simulink model "T2_simulation_2020a"  (R2022a)
settings: Solver=VariableStepAuto  StartTime=0.0  StopTime=simTime  RelTol=1e-3
values from neighbouring files (symbols this model uses):
  C11 = -0.1    [T2_PreLoadFcn.m]
  C21 = -0.1    [T2_PreLoadFcn.m]
undefined symbols (not defined in the file or in its folder): sysID_DAQ
libraries: cstblocks x1
settings Model: Creator=user
settings SolverCC: AlgebraicLoopSolver=TrustRegion
settings DataIOCC: ReturnWorkspaceOutputs=off
settings DebuggingCC: UnconnectedInputMsg=warning  UnconnectedOutputMsg=warning  UnconnectedLineMsg=warning  SFMachineParentedDataDiag=warning

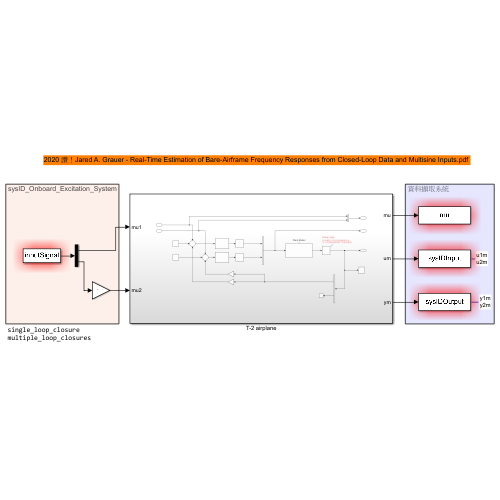
[thumbnail: Simulink's stored preview of the top-level diagram]
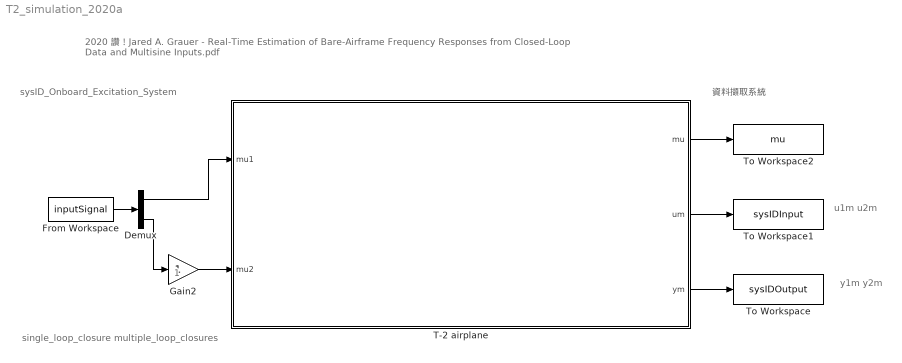
== system T2_simulation_2020a ==
  note: 1
  note: single_loop_closure
      | multiple_loop_closures
  note: sysID_Onboard_Excitation_System
  note: 資料擷取系統
  note: 2020 讚！Jared A. Grauer - Real-Time Estimation of Bare-Airframe Frequency Responses from Closed-Loop Data and Multisine Inputs.pdf
  note: u1m
      | u2m
  note: y1m
      | y2m
  Demux : Demux  Outputs=2
  From Workspace : FromWorkspace  VariableName=inputSignal  OutputAfterFinalValue=Holding final value
  Gain2 : Gain
  T-2 airplane : Subsystem
  To Workspace : ToWorkspace  VariableName=sysIDOutput  SaveFormat=Timeseries  SampleTime=sysID_DAQ.sampleTime
  To Workspace1 : ToWorkspace  VariableName=sysIDInput  SaveFormat=Timeseries  SampleTime=sysID_DAQ.sampleTime
  To Workspace2 : ToWorkspace  VariableName=mu  SaveFormat=Timeseries  SampleTime=sysID_DAQ.sampleTime
  wires:
  T-2 airplane/2(um) -> To Workspace1/1
  T-2 airplane/3(ym) -> To Workspace/1
  Gain2/1 -> T-2 airplane/2(mu2)
  Demux/2 -> Gain2/1
  Demux/1 -> T-2 airplane/1(mu1)
  From Workspace/1 -> Demux/1
  T-2 airplane/1(mu) -> To Workspace2/1

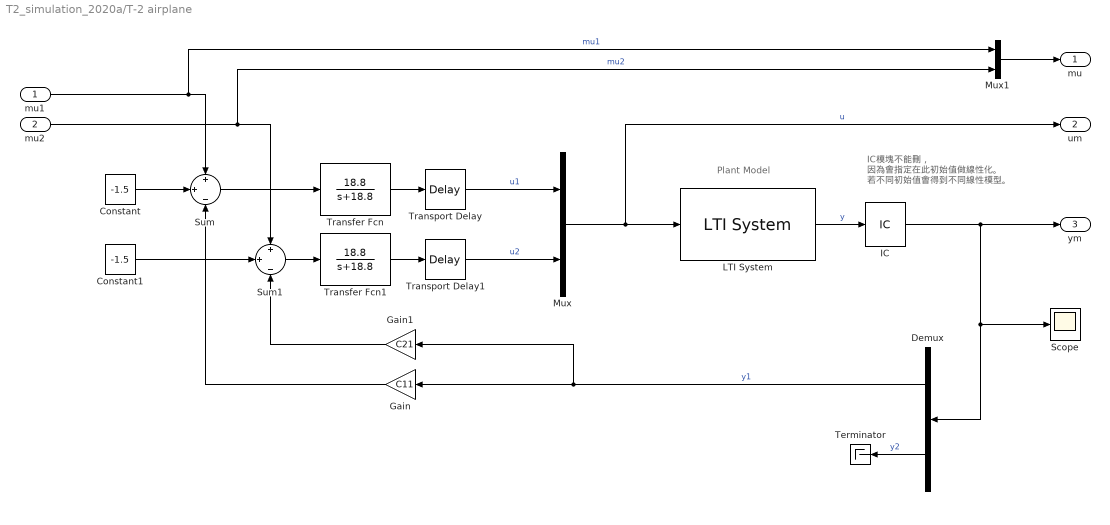
== system T2_simulation_2020a/T-2 airplane ==
  note: Plant Model
  note: IC模塊不能刪，
      | 因為會指定在此初始值做線性化。
      | 若不同初始值會得到不同線性模型。
  mu1 : Inport
  mu2 : Inport  Port=2
  Constant : Constant  Value=-1.5
  Constant1 : Constant  Value=-1.5
  Demux : Demux  Outputs=2
  Gain : Gain  Gain=C11
  Gain1 : Gain  Gain=C21
  IC : InitialCondition  Value=[0 -9.81]
  LTI System : cstblocks/LTI System  sys=sys  IC=[]
  Mux : Mux  Inputs=2
  Mux1 : Mux  Inputs=2
  Scope : Scope
  Sum : Sum  Inputs=+|+|-
  Sum1 : Sum  Inputs=+|+|-
  Terminator : Terminator
  Transfer Fcn : TransferFcn  Numerator=[18.8]  Denominator=[1 18.8]
  Transfer Fcn1 : TransferFcn  Numerator=[18.8]  Denominator=[1 18.8]
  Transport Delay : TransportDelay  DelayTime=0.01  InitialOutput=-1.5
  Transport Delay1 : TransportDelay  DelayTime=0.01  InitialOutput=-1.5
  mu : Outport
  um : Outport  Port=2
  ym : Outport  Port=3
  wires:
  Gain/1 -> Sum/3
  Gain1/1 -> Sum1/3
  Transfer Fcn/1 -> Transport Delay/1
  Constant1/1 -> Sum1/2
  Sum/1 -> Transfer Fcn/1
  Demux/1 -> Gain1/1, Gain/1  "y1"
  mu2/1 -> Mux1/2, Sum1/1  "mu2"
  Sum1/1 -> Transfer Fcn1/1
  LTI System/1 -> IC/1  "y"
  Transfer Fcn1/1 -> Transport Delay1/1
  Transport Delay1/1 -> Mux/2  "u2"
  Demux/2 -> Terminator/1  "y2"
  Transport Delay/1 -> Mux/1  "u1"
  Constant/1 -> Sum/2
  mu1/1 -> Mux1/1, Sum/1  "mu1"
  Mux/1 -> um/1, LTI System/1  "u"
  IC/1 -> ym/1, Scope/1, Demux/1
  Mux1/1 -> mu/1
